simulink model "logic"  (Simulink 6.6)
settings: Solver=FixedStepDiscrete  StartTime=0.0  StopTime=10.0  FixedStep=1  RelTol=1e-3
settings Model: Creator=hnine  LastModifiedBy=hnine

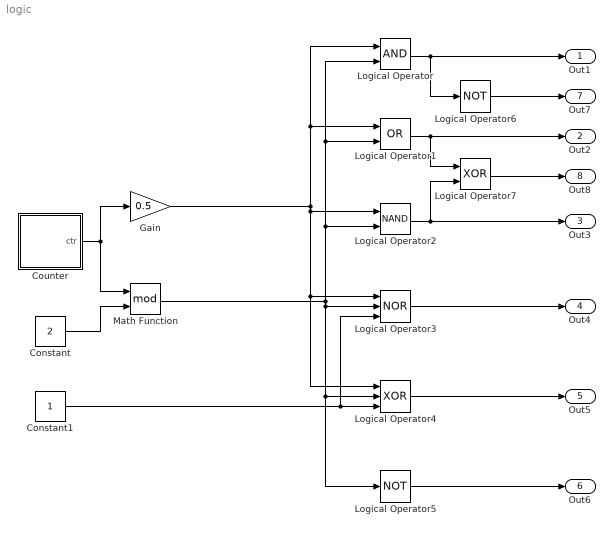
== system logic ==
  Constant : Constant  Value=2
  Constant1 : Constant
  Counter : Stateflow chart
  Gain : Gain  Gain=0.5  OutDataTypeMode=Specify via dialog  OutDataType=uint(16)
  Logical Operator : Logic  AllPortsSameDT=off  OutDataTypeMode=Boolean
  Logical Operator1 : Logic  Operator=OR  AllPortsSameDT=off  OutDataTypeMode=Boolean
  Logical Operator2 : Logic  Operator=NAND  AllPortsSameDT=off  OutDataTypeMode=Boolean
  Logical Operator3 : Logic  Operator=NOR  Inputs=3  AllPortsSameDT=off  OutDataTypeMode=Boolean
  Logical Operator4 : Logic  Operator=XOR  Inputs=3  AllPortsSameDT=off  OutDataTypeMode=Boolean
  Logical Operator5 : Logic  Operator=NOT  AllPortsSameDT=off  OutDataTypeMode=Boolean
  Logical Operator6 : Logic  Operator=NOT  AllPortsSameDT=off  OutDataTypeMode=Boolean
  Logical Operator7 : Logic  Operator=XOR  AllPortsSameDT=off  OutDataTypeMode=Boolean
  Math Function : Math  Operator=mod  SaturateOnIntegerOverflow=on
  Out1 : Outport
  Out2 : Outport  Port=2
  Out3 : Outport  Port=3
  Out4 : Outport  Port=4
  Out5 : Outport  Port=5
  Out6 : Outport  Port=6
  Out7 : Outport  Port=7
  Out8 : Outport  Port=8
  wires:
  Gain/1 -> Logical Operator4/1, Logical Operator3/1, Logical Operator/1, Logical Operator1/1, Logical Operator2/1
  Math Function/1 -> Logical Operator5/1, Logical Operator4/2, Logical Operator3/2, Logical Operator/2, Logical Operator1/2, Logical Operator2/2
  Logical Operator/1 -> Out1/1, Logical Operator6/1
  Logical Operator1/1 -> Out2/1, Logical Operator7/1
  Logical Operator2/1 -> Out3/1, Logical Operator7/2
  Logical Operator3/1 -> Out4/1
  Logical Operator4/1 -> Out5/1
  Logical Operator5/1 -> Out6/1
  Logical Operator6/1 -> Out7/1
  Counter/1(ctr) -> Gain/1, Math Function/1
  Constant/1 -> Math Function/2
  Logical Operator7/1 -> Out8/1
  Constant1/1 -> Logical Operator4/3, Logical Operator3/3

== stateflow chart Counter ==
  state s1
  (default) -> s1
  s1 -> s1 [order 1] : [ctr < 3] / ctr = ctr+1;
  s1 -> s1 [order 2] : [ctr >= 3] / ctr = 0;
  data: ctr output double =1
